simulink model "ground_test_EMF_new"  (R2024a)
settings: Solver=FixedStepAuto  StartTime=0.0  StopTime=0  FixedStep=framePeriod_s  RelTol=1e-3
undefined symbols (not defined in the file): Aircraft, aircraftIC, AircraftModel, Avphi, DiscIntNeverNeededParam, EMF, EnableFF, EnableRCHH, EnableSpeedHold, framePeriod_s, InitCond, Lv, Yv
libraries: simulink x13, simulink_extras x5
(part 2 of 3)

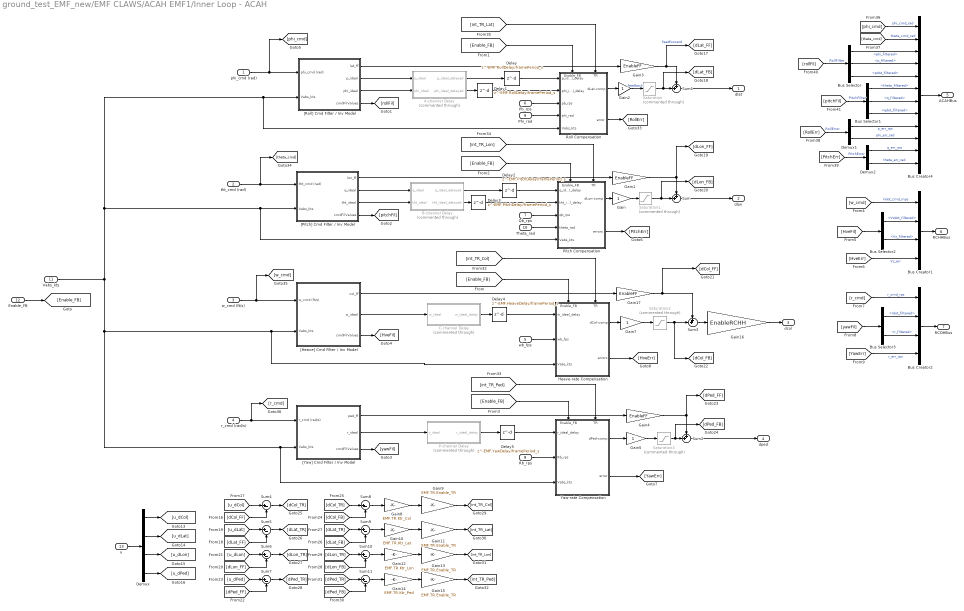
== system ground_test_EMF_new/EMF CLAWS/ACAH EMF1/Inner Loop - ACAH ==
  phi_cmd (rad) : Inport
  tht_cmd (rad) : Inport  Port=2
  w_cmd (ft/s) : Inport  Port=3
  r_cmd (rad/s) : Inport  Port=4
  wb_fps : Inport  Port=5
  Pb_rps : Inport  Port=6
  Qb_rps : Inport  Port=7
  Rb_rps : Inport  Port=8
  Phi_rad : Inport  Port=9
  Theta_rad : Inport  Port=10
  Vabs_kts : Inport  Port=11
  Enable_FB : Inport  Port=12
  u : Inport  Port=13
  A-channel Delay : Subsystem  Commented=through
  B-channel Delay : Subsystem  Commented=through
  Bus Creator1 : BusCreator  Inputs=4
  Bus Creator2 : BusCreator  Inputs=4
  Bus Creator4 : BusCreator  Inputs=12
  Bus Selector : BusSelector  OutputSignals=phi_filtered,p_filtered,pdot_filtered
  Bus Selector1 : BusSelector  OutputSignals=theta_filtered,q_filtered,qdot_filtered
  Bus Selector2 : BusSelector  OutputSignals=Vzdot_filtered,Vz_filtered
  Bus Selector3 : BusSelector  OutputSignals=rdot_filtered,r_filtered
  C-channel Delay : Subsystem  Commented=through
  Delay : Delay  DelayLength=EMF.RollDelay/framePeriod_s
  Delay1 : Delay  DelayLength=EMF.RollDelay/framePeriod_s
  Delay2 : Delay  DelayLength=EMF.PitchDelay/framePeriod_s
  Delay3 : Delay  DelayLength=EMF.PitchDelay/framePeriod_s
  Delay4 : Delay  DelayLength=EMF.HeaveDelay/framePeriod_s
  Delay5 : Delay  DelayLength=EMF.YawDelay/framePeriod_s
  Demux : Demux
  Demux1 : Demux  Outputs=2
  Demux2 : Demux  Outputs=2
  Gain{,2,5,7} (4 alike) : Gain
  Gain{1,3..4,17} (4 alike) : Gain  Gain=EnableFF
  Gain10 : Gain  Gain=EMF.TR.Ktr_Lat
  Gain{9,11,13,15} (4 alike) : Gain  Gain=EMF.TR.Enable_TR
  Gain12 : Gain  Gain=EMF.TR.Ktr_Lon
  Gain14 : Gain  Gain=EMF.TR.Ktr_Ped
  Gain16 : Gain  Gain=EnableRCHH
  Gain8 : Gain  Gain=EMF.TR.Ktr_Col
  Heave-rate Compensation : Subsystem
      settings: PortSchema="{\"entries\":[{\"content\":{\"sides\":[{\"content\":{\"connectorIds\":[\"In1\",\"In2\",\"In3\"]},\"type\":\"ConnectorPlacement.EquallySpacedRectSide\",\"uuid\":\"7252c1f8-7fe3-4075-bb5e-c3f9f1883e70\"},{\"content\":{\"connectorIds\":[\"Out1\",\"Out2\"],\"side\":\"RIGHT\"},\"type\":\"ConnectorPlacement.EquallySpacedRectSide\",\"uuid\":\"3c35276a-72f6-40d6-83e0-8018ffb9b035\"},{\"content\":{\"connectorIds\":[\"In4\",\"In5\"],\"side\":\"TOP\"},\"type\":\"ConnectorPlacement.EquallySpacedRectSide\",\"uuid\":\"6ce22a11-3d6f-44d3-856f-73f158445266\"}]},\"type\":\"ConnectorPlacement.EquallySpacedConnector\",\"uuid\":\"443ffc0d-1192-4812-a7f7-f46c9ac66e90\"}],\"packageUris\":[\"http://schema.mathworks.com/mf0/Connector/R2020b\"],\"version\":\"1.0\"}"
  P-channel Delay : Subsystem  Commented=through
  Pitch Compensation : Subsystem
      settings: PortSchema="{\"entries\":[{\"content\":{\"sides\":[{\"content\":{\"connectorIds\":[\"In1\",\"In2\",\"In3\",\"In4\",\"In5\"]},\"type\":\"ConnectorPlacement.EquallySpacedRectSide\",\"uuid\":\"45916f42-37ac-4154-8414-b45309659ed0\"},{\"content\":{\"connectorIds\":[\"Out1\",\"Out2\"],\"side\":\"RIGHT\"},\"type\":\"ConnectorPlacement.EquallySpacedRectSide\",\"uuid\":\"89f52b07-9cdc-4229-907e-581f3d5d6e1b\"},{\"content\":{\"connectorIds\":[\"In6\",\"In7\"],\"side\":\"TOP\"},\"type\":\"ConnectorPlacement.EquallySpacedRectSide\",\"uuid\":\"5e1074eb-2cc8-4130-bee4-0f8c72f9550d\"}]},\"type\":\"ConnectorPlacement.EquallySpacedConnector\",\"uuid\":\"11c4fb04-7926-4153-b42d-1368c1a6596f\"}],\"packageUris\":[\"http://schema.mathworks.com/mf0/Connector/R2020b\"],\"version\":\"1.0\"}"
  Roll Compensation : Subsystem
      settings: PortSchema="{\"entries\":[{\"content\":{\"sides\":[{\"content\":{\"connectorIds\":[\"In1\",\"In2\",\"In3\",\"In4\",\"In5\"]},\"type\":\"ConnectorPlacement.EquallySpacedRectSide\",\"uuid\":\"45916f42-37ac-4154-8414-b45309659ed0\"},{\"content\":{\"connectorIds\":[\"Out1\",\"Out2\"],\"side\":\"RIGHT\"},\"type\":\"ConnectorPlacement.EquallySpacedRectSide\",\"uuid\":\"89f52b07-9cdc-4229-907e-581f3d5d6e1b\"},{\"content\":{\"connectorIds\":[\"In6\",\"In7\"],\"side\":\"TOP\"},\"type\":\"ConnectorPlacement.EquallySpacedRectSide\",\"uuid\":\"5e1074eb-2cc8-4130-bee4-0f8c72f9550d\"}]},\"type\":\"ConnectorPlacement.EquallySpacedConnector\",\"uuid\":\"11c4fb04-7926-4153-b42d-1368c1a6596f\"}],\"packageUris\":[\"http://schema.mathworks.com/mf0/Connector/R2020b\"],\"version\":\"1.0\"}"
  Saturation : Saturate  Commented=through  UpperLimit=EMF.MaxCmd.pdot/2  LowerLimit=-EMF.MaxCmd.pdot/2
  Saturation1 : Saturate  Commented=through  UpperLimit=EMF.MaxCmd.qdot/2  LowerLimit=-EMF.MaxCmd.qdot/2
  Saturation2 : Saturate  Commented=through  UpperLimit=EMF.MaxCmd.wdot/2  LowerLimit=-EMF.MaxCmd.wdot/2
  Saturation3 : Saturate  Commented=through  UpperLimit=EMF.MaxCmd.rdot/2  LowerLimit=-EMF.MaxCmd.rdot/2
  Sum{,1..3} (4 alike) : Sum  Inputs=++|
  Sum{4..11} (8 alike) : Sum  Inputs=|+-
  Yaw-rate Compensation : Subsystem
      settings: PortSchema="{\"entries\":[{\"content\":{\"sides\":[{\"content\":{\"connectorIds\":[\"In1\",\"In2\",\"In3\"]},\"type\":\"ConnectorPlacement.EquallySpacedRectSide\",\"uuid\":\"7252c1f8-7fe3-4075-bb5e-c3f9f1883e70\"},{\"content\":{\"connectorIds\":[\"Out1\",\"Out2\"],\"side\":\"RIGHT\"},\"type\":\"ConnectorPlacement.EquallySpacedRectSide\",\"uuid\":\"3c35276a-72f6-40d6-83e0-8018ffb9b035\"},{\"content\":{\"connectorIds\":[\"In4\",\"In5\"],\"side\":\"TOP\"},\"type\":\"ConnectorPlacement.EquallySpacedRectSide\",\"uuid\":\"6ce22a11-3d6f-44d3-856f-73f158445266\"}]},\"type\":\"ConnectorPlacement.EquallySpacedConnector\",\"uuid\":\"443ffc0d-1192-4812-a7f7-f46c9ac66e90\"}],\"packageUris\":[\"http://schema.mathworks.com/mf0/Connector/R2020b\"],\"version\":\"1.0\"}"
  "[Heave] Cmd Filter / Inv Model" : Subsystem
  "[Pitch] Cmd Filter / Inv Model" : Subsystem
  "[Roll] Cmd Filter / Inv Model" : Subsystem
  "[Yaw] Cmd Filter / Inv Model" : Subsystem
  dlat : Outport
  dlon : Outport  Port=2
  dcol : Outport  Port=3
  dped : Outport  Port=4
  ACAHBus : Outport  Port=5
  RCHHBus : Outport  Port=6
  RCDHBus : Outport  Port=7
  wires:
  Gain17/1 -> [dCol_FF], Sum3/1
  Gain5/1 -> Saturation3/1
  Gain4/1 -> Sum2/1, [dPed_FF]
  Gain3/1 -> [dLat_FF], Sum1/1  "feedforward"
  Gain2/1 -> Saturation/1  "feedback"
  Gain1/1 -> [dLon_FF], Sum/1
  Gain/1 -> Saturation1/1
  wb_fps/1 -> Heave-rate Compensation/2(wb_fps)
  Rb_rps/1 -> Yaw-rate Compensation/2(Rb_rps)
  Theta_rad/1 -> Pitch Compensation/4(theta_rad)
  Qb_rps/1 -> Pitch Compensation/3(qb_rps)
  Phi_rad/1 -> Roll Compensation/4(phi_rad)
  Pb_rps/1 -> Roll Compensation/3(pb_rps)
  "[Roll] Cmd Filter / Inv Model"/1(lat_ff) -> Gain3/1
  Roll Compensation/1(dLat-comp) -> Gain2/1
  "[Pitch] Cmd Filter / Inv Model"/1(lon_ff) -> Gain1/1
  Pitch Compensation/1(dLon-comp) -> Gain/1
  w_cmd (ft/s)/1 -> [w_cmd], "[Heave] Cmd Filter / Inv Model"/1(w_cmd (ft/s))
  r_cmd (rad/s)/1 -> [r_cmd], "[Yaw] Cmd Filter / Inv Model"/1(r_cmd (rad/s))
  "[Yaw] Cmd Filter / Inv Model"/1(ped_ff) -> Gain4/1
  "[Heave] Cmd Filter / Inv Model"/1(col_ff) -> Gain17/1
  Yaw-rate Compensation/1(dPed-comp) -> Gain5/1
  Heave-rate Compensation/1(dCol-comp) -> Gain7/1
  Pitch Compensation/2(errors) -> [PitchErr]
  Yaw-rate Compensation/2(error) -> [YawErr]
  Heave-rate Compensation/2(errors) -> [HveErr]
  "[Heave] Cmd Filter / Inv Model"/3(cmdFilValues) -> [HveFil]
  "[Yaw] Cmd Filter / Inv Model"/3(cmdFilValues) -> [yawFil]
  "[Pitch] Cmd Filter / Inv Model"/4(cmdFilValues) -> [pitchFil]
  "[Roll] Cmd Filter / Inv Model"/4(cmdFilValues) -> [rollFil]
  C-channel Delay/1(w_ideal_delay) -> Delay4/1
  Sum3/1 -> Gain16/1
  "[Heave] Cmd Filter / Inv Model"/2(w_ideal) -> C-channel Delay/1(w_ideal)
  "[Yaw] Cmd Filter / Inv Model"/2(r_ideal) -> P-channel Delay/1(r_ideal)
  Sum2/1 -> dped/1
  P-channel Delay/1(r_ideal_delay) -> Delay5/1
  "[Roll] Cmd Filter / Inv Model"/3(phi_ideal) -> A-channel Delay/2(phi_ideal)
  Sum1/1 -> dlat/1
  "[Roll] Cmd Filter / Inv Model"/2(p_ideal) -> A-channel Delay/1(p_ideal)
  A-channel Delay/2(phi_ideal_delayed) -> Delay1/1
  A-channel Delay/1(p_ideal_delayed) -> Delay/1
  Sum/1 -> dlon/1
  B-channel Delay/2(tht_ideal_delayed) -> Delay3/1
  B-channel Delay/1(q_ideal_delayed) -> Delay2/1
  "[Pitch] Cmd Filter / Inv Model"/2(q_ideal) -> B-channel Delay/1(q_ideal)
  "[Pitch] Cmd Filter / Inv Model"/3(tht_ideal) -> B-channel Delay/2(tht_ideal)
  Vabs_kts/1 -> Heave-rate Compensation/3(Vabs_kts), "[Heave] Cmd Filter / Inv Model"/2(Vabs_kts), Yaw-rate Compensation/3(Vabs_kts), "[Yaw] Cmd Filter / Inv Model"/2(Vabs_kts), Pitch Compensation/5(Vabs_kts), "[Pitch] Cmd Filter / Inv Model"/2(Vabs_kts), Roll Compensation/5(Vabs_kts), "[Roll] Cmd Filter / Inv Model"/2(Vabs_kts)
  phi_cmd (rad)/1 -> [phi_cmd], "[Roll] Cmd Filter / Inv Model"/1(phi_cmd (rad))
  tht_cmd (rad)/1 -> [theta_cmd], "[Pitch] Cmd Filter / Inv Model"/1(tht_cmd (rad))
  Delay1/1 -> Roll Compensation/2(phi_ideal_delay)
  Delay/1 -> Roll Compensation/1(p_ideal_delay)
  Delay3/1 -> Pitch Compensation/2(tht_ideal_delay)
  Delay2/1 -> Pitch Compensation/1(q_ideal_delay)
  Delay4/1 -> Heave-rate Compensation/1(w_ideal_delay)
  Delay5/1 -> Yaw-rate Compensation/1(r_ideal_delay)
  Enable_FB/1 -> [Enable_FB]
  [Enable_FB] -> Heave-rate Compensation/4(Enable_FB)
  [Enable_FB] -> Roll Compensation/6(Enable_FB)
  [Enable_FB] -> Pitch Compensation/6(Enable_FB)
  [Enable_FB] -> Yaw-rate Compensation/4(Enable_FB)
  Gain7/1 -> Saturation2/1
  Saturation/1 -> [dLat_FB], Sum1/2
  Saturation1/1 -> [dLon_FB], Sum/2
  Saturation3/1 -> [dPed_FB], Sum2/2
  u/1 -> Demux/1
  Demux/1 -> [u_dCol]
  Demux/4 -> [u_dPed]
  Demux/3 -> [u_dLon]
  Demux/2 -> [u_dLat]
  [u_dCol] -> Sum4/1
  [dCol_FF] -> Sum4/2
  Sum4/1 -> [dCol_TR]
  Sum5/1 -> [dLat_TR]
  [dLat_FF] -> Sum5/2
  [u_dLat] -> Sum5/1
  [u_dLon] -> Sum6/1
  [dLon_FF] -> Sum6/2
  Sum6/1 -> [dLon_TR]
  Sum7/1 -> [dPed_TR]
  [dPed_FF] -> Sum7/2
  [u_dPed] -> Sum7/1
  Sum8/1 -> Gain8/1
  [dCol_FB] -> Sum8/2
  [dCol_TR] -> Sum8/1
  Gain8/1 -> Gain9/1
  Gain9/1 -> [int_TR_Col]
  Gain11/1 -> [int_TR_Lat]
  Gain10/1 -> Gain11/1
  [dLat_TR] -> Sum9/1
  [dLat_FB] -> Sum9/2
  Sum9/1 -> Gain10/1
  Sum10/1 -> Gain12/1
  [dLon_FB] -> Sum10/2
  [dLon_TR] -> Sum10/1
  Gain12/1 -> Gain13/1
  Gain13/1 -> [int_TR_Lon]
  Gain15/1 -> [int_TR_Ped]
  Gain14/1 -> Gain15/1
  [dPed_TR] -> Sum11/1
  [dPed_FB] -> Sum11/2
  Sum11/1 -> Gain14/1
  [int_TR_Col] -> Heave-rate Compensation/5(TR)
  [int_TR_Ped] -> Yaw-rate Compensation/5(TR)
  [int_TR_Lon] -> Pitch Compensation/7(TR)
  [int_TR_Lat] -> Roll Compensation/7(TR)
  Saturation2/1 -> [dCol_FB], Sum3/2
  Gain16/1 -> dcol/1
  Roll Compensation/2(error) -> [RollErr]
  Bus Creator4/1 -> ACAHBus/1
  [phi_cmd] -> Bus Creator4/1  "phi_cmd_rad"
  [theta_cmd] -> Bus Creator4/2  "theta_cmd_rad"
  [rollFil] -> Bus Selector/1  "RollFilter"
  [pitchFil] -> Bus Selector1/1  "PitchFilter"
  Bus Selector/2 -> Bus Creator4/4  "<p_filtered>"
  Bus Selector/1 -> Bus Creator4/3  "<phi_filtered>"
  Bus Selector/3 -> Bus Creator4/5  "<pdot_filtered>"
  Bus Selector1/1 -> Bus Creator4/6  "<theta_filtered>"
  Bus Selector1/2 -> Bus Creator4/7  "<q_filtered>"
  Bus Selector1/3 -> Bus Creator4/8  "<qdot_filtered>"
  [RollErr] -> Demux1/1  "RollError"
  [PitchErr] -> Demux2/1  "PitchError"
  Demux2/2 -> Bus Creator4/12  "theta_err_rad"
  Demux2/1 -> Bus Creator4/11  "q_err_rps"
  Demux1/1 -> Bus Creator4/9  "p_err_rps"
  Demux1/2 -> Bus Creator4/10  "phi_err_rad"
  Bus Creator1/1 -> RCHHBus/1
  [w_cmd] -> Bus Creator1/1  "hdot_cmd_mps"
  [HveFil] -> Bus Selector2/1
  Bus Selector2/2 -> Bus Creator1/3  "<Vz_filtered>"
  Bus Selector2/1 -> Bus Creator1/2  "<Vzdot_filtered>"
  [HveErr] -> Bus Creator1/4  "Vz_err"
  [YawErr] -> Bus Creator2/4  "r_err_rps"
  Bus Selector3/1 -> Bus Creator2/2  "<rdot_filtered>"
  Bus Selector3/2 -> Bus Creator2/3  "<r_filtered>"
  [yawFil] -> Bus Selector3/1
  [r_cmd] -> Bus Creator2/1  "r_cmd_rps"
  Bus Creator2/1 -> RCDHBus/1

== system ground_test_EMF_new/EMF CLAWS/ACAH EMF1/Mixer ==
  ControlMoments : Inport
  Constant : Constant  Value=EMF.Mixer(:,:,1)
  Matrix Multiply : Product  Multiplication=Matrix(*)
  Rotor Speeds : Outport
  wires:
  Constant/1 -> Matrix Multiply/1
  ControlMoments/1 -> Matrix Multiply/2
  Matrix Multiply/1 -> Rotor Speeds/1  "Rotor Speeds"

== system ground_test_EMF_new/EMF CLAWS/ACAH EMF1/OnGroundController ==
  cmdsACT : Inport
  Get ACAH Commands1 : Subsystem
      settings: PortSchema="{\"entries\":[{\"content\":{\"sides\":[{\"content\":{\"connectorIds\":[\"In1\"]},\"type\":\"ConnectorPlacement.EquallySpacedRectSide\",\"uuid\":\"7c65b894-e97e-426b-b3a6-5e2b2b7aa780\"},{\"content\":{\"connectorIds\":[\"Out1\"],\"side\":\"RIGHT\"},\"type\":\"ConnectorPlacement.EquallySpacedRectSide\",\"uuid\":\"da5e6856-a2cd-4302-9f49-e9c1cc422564\"},{\"content\":{\"connectorIds\":[\"Out2\"],\"side\":\"TOP\"},\"type\":\"ConnectorPlacement.EquallySpacedRectSide\",\"uuid\":\"a744aea1-4523-47bd-90bf-604bddb972da\"}]},\"type\":\"ConnectorPlacement.EquallySpacedConnector\",\"uuid\":\"254b2f3c-23c2-4cd5-a42e-cd931c0875f5\"}],\"packageUris\":[\"http://schema.mathworks.com/mf0/Connector/R2020b\"],\"version\":\"1.0\"}"
  OL rotor speeds from throttle : Subsystem  Commented=through
  TrimOmegas_OL : Outport
  CmdMoments_Ground : Outport  Port=2
  wires:
  cmdsACT/1 -> Get ACAH Commands1/1(StickInputs)
  Get ACAH Commands1/1(cmdsACAH) -> CmdMoments_Ground/1
  Get ACAH Commands1/2(throttleOmega) -> OL rotor speeds from throttle/1(throttleOmega)
  OL rotor speeds from throttle/1(Omegas_rps) -> TrimOmegas_OL/1

== system ground_test_EMF_new/EMF CLAWS/ACAH EMF1/Rate Saturation ==
  dlat : Inport
  dlon : Inport  Port=2
  dcol : Inport  Port=3
  dped : Inport  Port=4
  Compare To Constant1 : simulink/Logic and Bit Operations/Compare To Constant  relop=<  const=-EMF.MaxCmd.qdot  OutDataTypeStr=boolean
  Compare To Constant2 : simulink/Logic and Bit Operations/Compare To Constant  relop=>  const=EMF.MaxCmd.qdot  OutDataTypeStr=boolean
  Compare To Constant3 : simulink/Logic and Bit Operations/Compare To Constant  relop=<  const=-EMF.MaxCmd.wdot  OutDataTypeStr=boolean
  Compare To Constant4 : simulink/Logic and Bit Operations/Compare To Constant  relop=>  const=EMF.MaxCmd.wdot  OutDataTypeStr=boolean
  Compare To Constant5 : simulink/Logic and Bit Operations/Compare To Constant  relop=<  const=-EMF.MaxCmd.rdot  OutDataTypeStr=boolean
  Compare To Constant6 : simulink/Logic and Bit Operations/Compare To Constant  relop=>  const=EMF.MaxCmd.rdot  OutDataTypeStr=boolean
  Compare To Constant7 : simulink/Logic and Bit Operations/Compare To Constant  relop=<  const=-EMF.MaxCmd.pdot  OutDataTypeStr=boolean
  Compare To Constant8 : simulink/Logic and Bit Operations/Compare To Constant  relop=>  const=EMF.MaxCmd.pdot  OutDataTypeStr=boolean
  Logical Operator{1..4} (4 alike) : Logic  Operator=OR  AllPortsSameDT=off  OutDataTypeStr=boolean
  Mux : Mux
  Saturation : Saturate  UpperLimit=EMF.MaxCmd.pdot  LowerLimit=-EMF.MaxCmd.pdot
  Saturation1 : Saturate  UpperLimit=EMF.MaxCmd.qdot  LowerLimit=-EMF.MaxCmd.qdot
  Saturation2 : Saturate  UpperLimit=EMF.MaxCmd.wdot  LowerLimit=-EMF.MaxCmd.wdot
  Saturation3 : Saturate  UpperLimit=EMF.MaxCmd.rdot  LowerLimit=-EMF.MaxCmd.rdot
  dcol sat : Outport
  dlat sat : Outport  Port=2
  dlon sat : Outport  Port=3
  dped sat : Outport  Port=4
  Flag : Outport  Port=5
  wires:
  Saturation3/1 -> dped sat/1
  Saturation1/1 -> dlon sat/1
  Saturation/1 -> dlat sat/1
  dlat/1 -> Compare To Constant8/1, Compare To Constant7/1, Saturation/1
  Saturation2/1 -> dcol sat/1
  Compare To Constant7/1 -> Logical Operator4/2
  Compare To Constant8/1 -> Logical Operator4/1
  Logical Operator4/1 -> Mux/1
  Logical Operator1/1 -> Mux/2
  Compare To Constant2/1 -> Logical Operator1/1
  Compare To Constant1/1 -> Logical Operator1/2
  dlon/1 -> Compare To Constant2/1, Compare To Constant1/1, Saturation1/1
  dcol/1 -> Compare To Constant3/1, Compare To Constant4/1, Saturation2/1
  Compare To Constant3/1 -> Logical Operator2/2
  Compare To Constant4/1 -> Logical Operator2/1
  Logical Operator2/1 -> Mux/3
  Logical Operator3/1 -> Mux/4
  Compare To Constant6/1 -> Logical Operator3/1
  Compare To Constant5/1 -> Logical Operator3/2
  dped/1 -> Saturation3/1, Compare To Constant6/1, Compare To Constant5/1
  Mux/1 -> Flag/1

== system ground_test_EMF_new/EMF CLAWS/ACAH EMF1/Remap Rotor Speeds to PWM ==
  Rotor Speeds : Inport
  Constant1 : Constant  Value=AircraftModel.MinOmegaLimit
  Constant2 : Constant  Value=AircraftModel.MaxOmegaLimit
  Constant3 : Constant  Value=AircraftModel.MinPWMLimit*ones(1,4)
  Constant4 : Constant  Value=AircraftModel.MaxPWMLimit*ones(4,1)
  Rotor Speed Saturation : Subsystem
  remap : MATLAB Function  TreatAsAtomicUnit=on
  PWM_int16 : Outport
  tag scope: OmSatFlag=global
  wires:
  Rotor Speed Saturation/2(Saturated Rotor Speeds) -> remap/1(norm_in)
  Rotor Speed Saturation/1(OmegaSaturationFlags) -> [OmSatFlag]
  Constant2/1 -> remap/3(in_max)
  remap/1(raw_out) -> PWM_int16/1  "PWM_cont"
  Constant4/1 -> remap/5(out_max)
  Constant1/1 -> remap/2(in_min)
  Constant3/1 -> remap/4(out_min)
  Rotor Speeds/1 -> Rotor Speed Saturation/1(Rotor Speeds)

== system ground_test_EMF_new/EMF CLAWS/ACAH EMF1/Subsystem ==
  StateBus : Inport
  Add : Sum  Inputs=+++
  Bus Selector1 : BusSelector  OutputSignals=u_fdbk_mps,v_fdbk_mps,w_fdbk_mps
  Gain : Gain  Gain=0
  Sqrt : Sqrt
  Square : Math  Operator=square
  Square1 : Math  Operator=square
  Square2 : Math  Operator=square
  fps_to_kts : Gain  Gain=0.592484
  Vabs_kts : Outport
  wires:
  Square1/1 -> Add/2
  Bus Selector1/3 -> Square2/1  "<w_fdbk_mps>"
  StateBus/1 -> Bus Selector1/1
  Add/1 -> Sqrt/1
  Square/1 -> Add/1
  Bus Selector1/1 -> Square/1  "<u_fdbk_mps>"
  Bus Selector1/2 -> Gain/1  "<v_fdbk_mps>"
  Sqrt/1 -> fps_to_kts/1
  Square2/1 -> Add/3
  Gain/1 -> Square1/1
  fps_to_kts/1 -> Vabs_kts/1

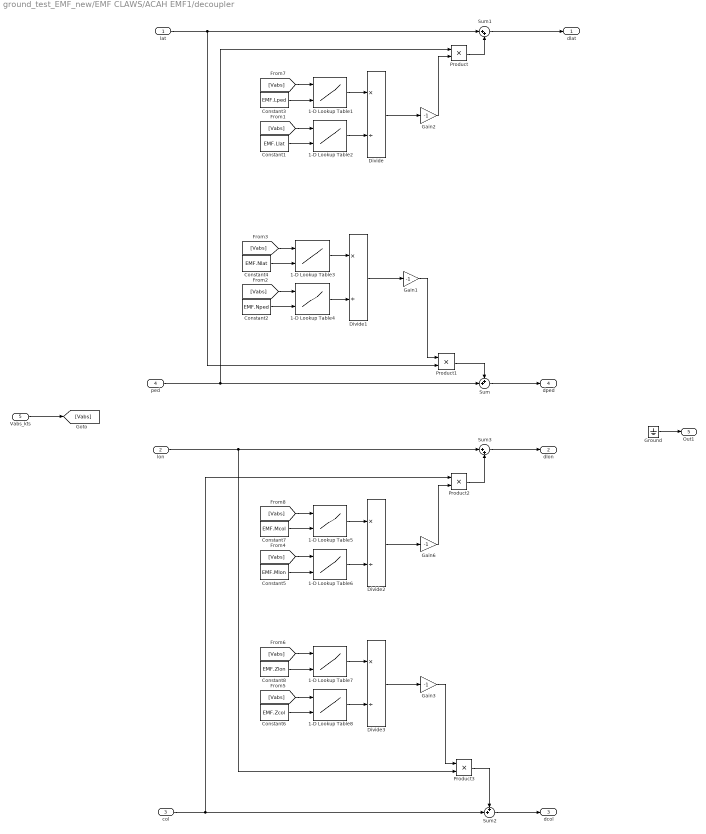
== system ground_test_EMF_new/EMF CLAWS/ACAH EMF1/decoupler ==
  lat : Inport
  lon : Inport  Port=2
  col : Inport  Port=3
  ped : Inport  Port=4
  Vabs_kts : Inport  Port=5
  1-D Lookup Table{1..8} (8 alike) : Lookup_n-D  NumberOfTableDimensions=1  BreakpointsForDimension1=EMF.VTAB  BeginIndexSearchUsingPreviousIndexResult=on  TableSource=Input port  Table=tanh([-5:5])  ExtrapMethod=Clip  InternalRulePriority=Speed  RndMeth=Simplest
      settings: InputPortMap=u0,p221
  Constant1 : Constant  Value=EMF.Llat
  Constant2 : Constant  Value=EMF.Nped
  Constant3 : Constant  Value=EMF.Lped
  Constant4 : Constant  Value=EMF.Nlat
  Constant5 : Constant  Value=EMF.Mlon
  Constant6 : Constant  Value=EMF.Zcol
  Constant7 : Constant  Value=EMF.Mcol
  Constant8 : Constant  Value=EMF.Zlon
  Divide{,1..3} (4 alike) : Product  Inputs=*/
  Gain{1..3,6} (4 alike) : Gain  Gain=-1
  Ground : Ground
  Product{,1..3} (4 alike) : Product
  Sum : Sum  Inputs=++|
  Sum1 : Sum  Inputs=|++
  Sum2 : Sum  Inputs=++|
  Sum3 : Sum  Inputs=|++
  dlat : Outport
  dlon : Outport  Port=2
  dcol : Outport  Port=3
  dped : Outport  Port=4
  Out1 : Outport  Port=5
  wires:
  Vabs_kts/1 -> [Vabs]
  Product3/1 -> Sum2/1
  Product2/1 -> Sum3/2
  Constant7/1 -> 1-D Lookup Table5/2
  [Vabs] -> 1-D Lookup Table5/1
  [Vabs] -> 1-D Lookup Table6/1
  Constant5/1 -> 1-D Lookup Table6/2
  1-D Lookup Table6/1 -> Divide2/2
  1-D Lookup Table5/1 -> Divide2/1
  Divide2/1 -> Gain6/1
  Gain6/1 -> Product2/2
  Gain3/1 -> Product3/1
  Divide3/1 -> Gain3/1
  1-D Lookup Table7/1 -> Divide3/1
  1-D Lookup Table8/1 -> Divide3/2
  Constant6/1 -> 1-D Lookup Table8/2
  [Vabs] -> 1-D Lookup Table8/1
  [Vabs] -> 1-D Lookup Table7/1
  Constant8/1 -> 1-D Lookup Table7/2
  Product1/1 -> Sum/1
  Constant4/1 -> 1-D Lookup Table3/2
  [Vabs] -> 1-D Lookup Table3/1
  [Vabs] -> 1-D Lookup Table4/1
  Constant2/1 -> 1-D Lookup Table4/2
  1-D Lookup Table4/1 -> Divide1/2
  1-D Lookup Table3/1 -> Divide1/1
  Divide1/1 -> Gain1/1
  Gain1/1 -> Product1/1
  Gain2/1 -> Product/2
  Product/1 -> Sum1/2
  Divide/1 -> Gain2/1
  1-D Lookup Table1/1 -> Divide/1
  1-D Lookup Table2/1 -> Divide/2
  Constant1/1 -> 1-D Lookup Table2/2
  [Vabs] -> 1-D Lookup Table2/1
  [Vabs] -> 1-D Lookup Table1/1
  Constant3/1 -> 1-D Lookup Table1/2
  Sum3/1 -> dlon/1
  Sum2/1 -> dcol/1
  Sum1/1 -> dlat/1
  ped/1 -> Sum/2, Product/1
  lat/1 -> Sum1/1, Product1/2
  Sum/1 -> dped/1
  col/1 -> Product2/1, Sum2/2
  lon/1 -> Product3/2, Sum3/1
  Ground/1 -> Out1/1

== system ground_test_EMF_new/EMF CLAWS/ACAH EMF1/Inner Loop - ACAH/A-channel Delay ==
  p_ideal : Inport
  phi_ideal : Inport  Port=2
  Constant : Constant  Value=EMF.tauf
  Demux : Demux  Outputs=2
  Divide : Product  Inputs=*/
  Integrator : Integrator
  Mux : Mux  Inputs=2
  Sum : Sum  Inputs=|+-
  p_ideal_delayed : Outport
  phi_ideal_delayed : Outport  Port=2
  wires:
  Demux/2 -> phi_ideal_delayed/1
  Demux/1 -> p_ideal_delayed/1
  phi_ideal/1 -> Mux/2
  p_ideal/1 -> Mux/1
  Mux/1 -> Sum/1
  Constant/1 -> Divide/2
  Divide/1 -> Integrator/1
  Sum/1 -> Divide/1
  Integrator/1 -> Demux/1, Sum/2

== system ground_test_EMF_new/EMF CLAWS/ACAH EMF1/Inner Loop - ACAH/B-channel Delay ==
  q_ideal : Inport
  tht_ideal : Inport  Port=2
  Constant : Constant  Value=EMF.tauf
  Demux : Demux  Outputs=2
  Divide : Product  Inputs=*/
  Integrator : Integrator
  Mux : Mux  Inputs=2
  Sum : Sum  Inputs=|+-
  q_ideal_delayed : Outport
  tht_ideal_delayed : Outport  Port=2
  wires:
  Demux/2 -> tht_ideal_delayed/1
  Demux/1 -> q_ideal_delayed/1
  tht_ideal/1 -> Mux/2
  q_ideal/1 -> Mux/1
  Mux/1 -> Sum/1
  Constant/1 -> Divide/2
  Divide/1 -> Integrator/1
  Sum/1 -> Divide/1
  Integrator/1 -> Demux/1, Sum/2

== system ground_test_EMF_new/EMF CLAWS/ACAH EMF1/Inner Loop - ACAH/C-channel Delay ==
  w_ideal : Inport
  Constant : Constant  Value=EMF.tauf
  Divide : Product  Inputs=*/
  Integrator : Integrator
  Sum : Sum  Inputs=|+-
  w_ideal_delay : Outport
  wires:
  w_ideal/1 -> Sum/1
  Constant/1 -> Divide/2
  Divide/1 -> Integrator/1
  Sum/1 -> Divide/1
  Integrator/1 -> w_ideal_delay/1, Sum/2

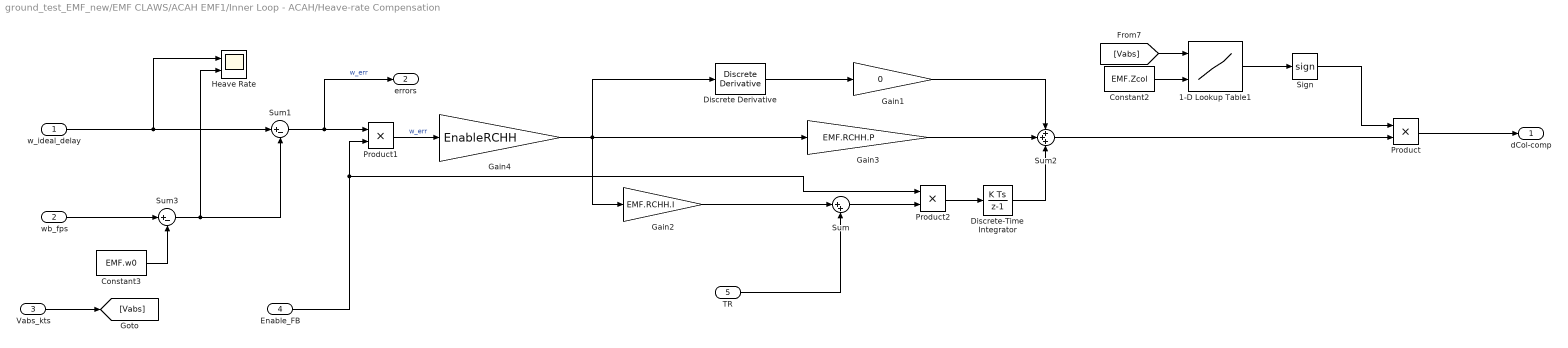
== system ground_test_EMF_new/EMF CLAWS/ACAH EMF1/Inner Loop - ACAH/Heave-rate Compensation ==
  w_ideal_delay : Inport
  wb_fps : Inport  Port=2
  Vabs_kts : Inport  Port=3
  Enable_FB : Inport  Port=4
  TR : Inport  Port=5
  1-D Lookup Table1 : Lookup_n-D  NumberOfTableDimensions=1  BreakpointsForDimension1=EMF.VTAB  BeginIndexSearchUsingPreviousIndexResult=on  TableSource=Input port  Table=tanh([-5:5])  ExtrapMethod=Clip  InternalRulePriority=Speed  RndMeth=Simplest
      settings: InputPortMap=u0,p221
  Constant2 : Constant  Value=EMF.Zcol
  Constant3 : Constant  Value=EMF.w0
  Discrete Derivative : simulink/Discrete/Discrete Derivative  gainval=1.0  ICPrevScaledInput=0.0  OutMin=[]  OutMax=[]  OutDataType=fixdt(1, 16)  OutScaling=2^-10  DoSatur=off
  Discrete-Time Integrator : DiscreteIntegrator  SampleTime=-1  ICPrevOutput=DiscIntNeverNeededParam  ICPrevScaledInput=DiscIntNeverNeededParam
  Gain1 : Gain  Gain=0
  Gain2 : Gain  Gain=EMF.RCHH.I
  Gain3 : Gain  Gain=EMF.RCHH.P
  Gain4 : Gain  Gain=EnableRCHH
  Heave Rate : Scope  NumInputPorts=2
  Product : Product
  Product1 : Product
  Product2 : Product
  Sign : Signum
  Sum : Sum  Inputs=|++
  Sum1 : Sum  Inputs=|+-
  Sum2 : Sum  Inputs=+++
  Sum3 : Sum  Inputs=|+-
  dCol-comp : Outport
  errors : Outport  Port=2
  wires:
  Gain3/1 -> Sum2/2
  Sum/1 -> Product2/2
  wb_fps/1 -> Sum3/1
  Sign/1 -> Product/1
  1-D Lookup Table1/1 -> Sign/1
  Product/1 -> dCol-comp/1
  Discrete Derivative/1 -> Gain1/1
  Product1/1 -> Gain4/1  "w_err"
  Sum2/1 -> Product/2
  Gain1/1 -> Sum2/1
  w_ideal_delay/1 -> Heave Rate/1, Sum1/1
  [Vabs] -> 1-D Lookup Table1/1
  Constant2/1 -> 1-D Lookup Table1/2
  Vabs_kts/1 -> [Vabs]
  Sum3/1 -> Heave Rate/2, Sum1/2
  Constant3/1 -> Sum3/2
  Sum1/1 -> errors/1, Product1/1  "w_err"
  Enable_FB/1 -> Product2/1, Product1/2
  Discrete-Time Integrator/1 -> Sum2/3
  Product2/1 -> Discrete-Time Integrator/1
  Gain2/1 -> Sum/1
  TR/1 -> Sum/2
  Gain4/1 -> Discrete Derivative/1, Gain3/1, Gain2/1

== system ground_test_EMF_new/EMF CLAWS/ACAH EMF1/Inner Loop - ACAH/P-channel Delay ==
  r_ideal : Inport
  Constant : Constant  Value=EMF.tauf
  Divide : Product  Inputs=*/
  Integrator : Integrator
  Sum : Sum  Inputs=|+-
  r_ideal_delay : Outport
  wires:
  Divide/1 -> Integrator/1
  r_ideal/1 -> Sum/1
  Integrator/1 -> Sum/2, r_ideal_delay/1
  Constant/1 -> Divide/2
  Sum/1 -> Divide/1

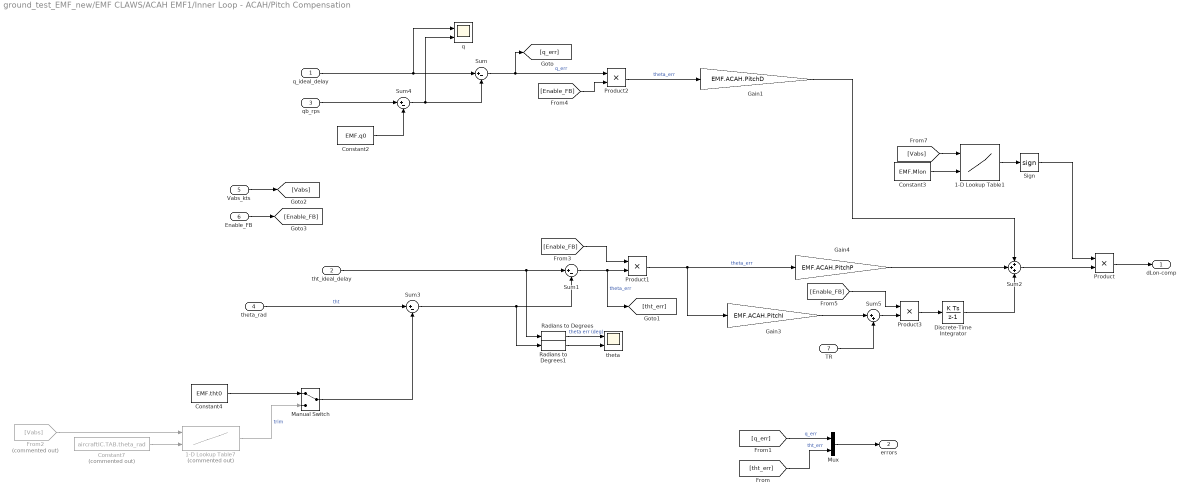
== system ground_test_EMF_new/EMF CLAWS/ACAH EMF1/Inner Loop - ACAH/Pitch Compensation ==
  q_ideal_delay : Inport
  tht_ideal_delay : Inport  Port=2
  qb_rps : Inport  Port=3
  theta_rad : Inport  Port=4
  Vabs_kts : Inport  Port=5
  Enable_FB : Inport  Port=6
  TR : Inport  Port=7
  1-D Lookup Table1 : Lookup_n-D  NumberOfTableDimensions=1  BreakpointsForDimension1=EMF.VTAB  BeginIndexSearchUsingPreviousIndexResult=on  TableSource=Input port  Table=tanh([-5:5])  ExtrapMethod=Clip  InternalRulePriority=Speed  RndMeth=Simplest
      settings: InputPortMap=u0,p221
  1-D Lookup Table7 : Lookup_n-D  Commented=on  NumberOfTableDimensions=1  BreakpointsForDimension1=EMF.VTAB  BeginIndexSearchUsingPreviousIndexResult=on  TableSource=Input port  Table=tanh([-5:5])  ExtrapMethod=Clip  InternalRulePriority=Speed  RndMeth=Simplest
      settings: InputPortMap=u0,p221
  Constant2 : Constant  Value=EMF.q0
  Constant3 : Constant  Value=EMF.Mlon
  Constant4 : Constant  Value=EMF.tht0
  Constant7 : Constant  Commented=on  Value=aircraftIC.TAB.theta_rad
  Discrete-Time Integrator : DiscreteIntegrator  SampleTime=-1  ICPrevOutput=DiscIntNeverNeededParam  ICPrevScaledInput=DiscIntNeverNeededParam
  From2 : From  Commented=on  GotoTag=Vabs
  Gain1 : Gain  Gain=EMF.ACAH.PitchD
  Gain3 : Gain  Gain=EMF.ACAH.PitchI
  Gain4 : Gain  Gain=EMF.ACAH.PitchP
  Manual Switch : ManualSwitch
  Mux : Mux  Inputs=2
  Product{,1..3} (4 alike) : Product
  Radians to Degrees : simulink_extras/Transformations/Radians to Degrees
  Radians to Degrees1 : simulink_extras/Transformations/Radians to Degrees
  Sign : Signum
  Sum{,1,3..4} (4 alike) : Sum  Inputs=|+-
  Sum2 : Sum  Inputs=+++
  Sum5 : Sum  Inputs=|++
  q : Scope  NumInputPorts=2
  theta : Scope  NumInputPorts=2
  dLon-comp : Outport
  errors : Outport  Port=2
  wires:
  Gain4/1 -> Sum2/2
  Sign/1 -> Product/1
  Product/1 -> dLon-comp/1
  Gain1/1 -> Sum2/1
  [q_err] -> Mux/1  "q_err"
  Mux/1 -> errors/1
  [tht_err] -> Mux/2  "tht_err"
  Sum/1 -> Product2/1, [q_err]  "q_err"
  Product1/1 -> Gain3/1, Gain4/1  "theta_err"
  q_ideal_delay/1 -> Sum/1, q/1
  qb_rps/1 -> Sum4/1
  Sum4/1 -> Sum/2, q/2
  Constant2/1 -> Sum4/2
  [Vabs] -> 1-D Lookup Table1/1
  Constant3/1 -> 1-D Lookup Table1/2
  1-D Lookup Table1/1 -> Sign/1
  Vabs_kts/1 -> [Vabs]
  Radians to Degrees/1 -> theta/1  "theta err (deg)"
  Radians to Degrees1/1 -> theta/2
  Constant7/1 -> 1-D Lookup Table7/2
  Constant4/1 -> Manual Switch/1
  Sum3/1 -> Sum1/2, Radians to Degrees1/1
  From2/1 -> 1-D Lookup Table7/1
  theta_rad/1 -> Sum3/1  "tht"
  1-D Lookup Table7/1 -> Manual Switch/2  "trim"
  Sum5/1 -> Product3/2
  tht_ideal_delay/1 -> Sum1/1, Radians to Degrees/1
  Sum2/1 -> Product/2
  Manual Switch/1 -> Sum3/2
  Sum1/1 -> [tht_err], Product1/2  "theta_err"
  Enable_FB/1 -> [Enable_FB]
  [Enable_FB] -> Product1/1
  Product2/1 -> Gain1/1  "theta_err"
  [Enable_FB] -> Product2/2
  Discrete-Time Integrator/1 -> Sum2/3
  Product3/1 -> Discrete-Time Integrator/1
  [Enable_FB] -> Product3/1
  Gain3/1 -> Sum5/1
  TR/1 -> Sum5/2

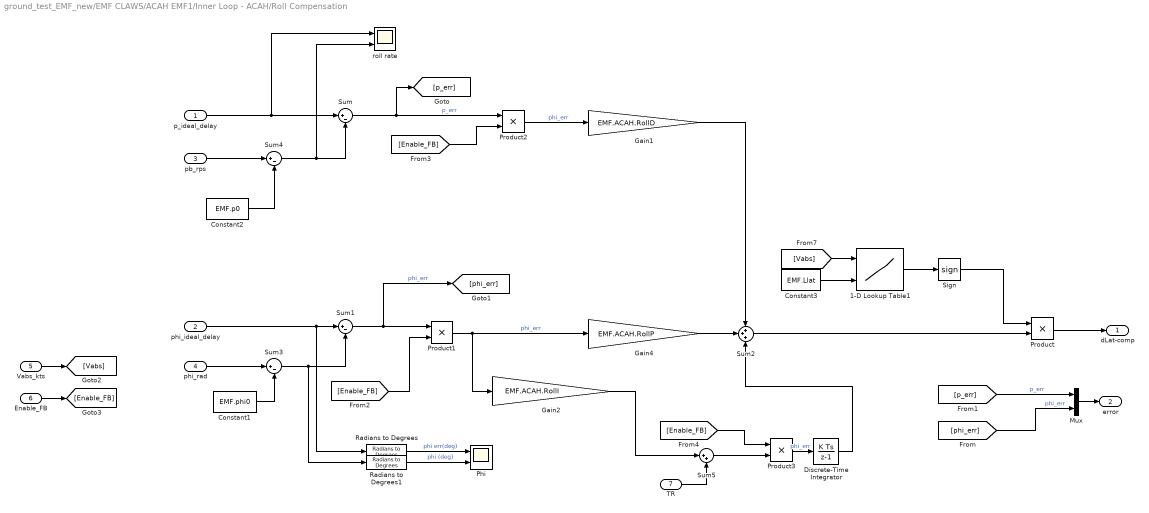
== system ground_test_EMF_new/EMF CLAWS/ACAH EMF1/Inner Loop - ACAH/Roll Compensation ==
  p_ideal_delay : Inport
  phi_ideal_delay : Inport  Port=2
  pb_rps : Inport  Port=3
  phi_rad : Inport  Port=4
  Vabs_kts : Inport  Port=5
  Enable_FB : Inport  Port=6
  TR : Inport  Port=7
  1-D Lookup Table1 : Lookup_n-D  NumberOfTableDimensions=1  BreakpointsForDimension1=EMF.VTAB  BeginIndexSearchUsingPreviousIndexResult=on  TableSource=Input port  Table=tanh([-5:5])  ExtrapMethod=Clip  InternalRulePriority=Speed  RndMeth=Simplest
      settings: InputPortMap=u0,p221
  Constant1 : Constant  Value=EMF.phi0
  Constant2 : Constant  Value=EMF.p0
  Constant3 : Constant  Value=EMF.Llat
  Discrete-Time Integrator : DiscreteIntegrator  SampleTime=-1  ICPrevOutput=DiscIntNeverNeededParam  ICPrevScaledInput=DiscIntNeverNeededParam
  Gain1 : Gain  Gain=EMF.ACAH.RollD
  Gain2 : Gain  Gain=EMF.ACAH.RollI
  Gain4 : Gain  Gain=EMF.ACAH.RollP
  Mux : Mux  Inputs=2
  Phi : Scope  NumInputPorts=2
  Product{,1..3} (4 alike) : Product
  Radians to Degrees : simulink_extras/Transformations/Radians to Degrees
  Radians to Degrees1 : simulink_extras/Transformations/Radians to Degrees
  Sign : Signum
  Sum{,1,3..4} (4 alike) : Sum  Inputs=|+-
  Sum2 : Sum  Inputs=+++
  Sum5 : Sum  Inputs=|++
  roll rate : Scope  NumInputPorts=2
  dLat-comp : Outport
  error : Outport  Port=2
  wires:
  Gain4/1 -> Sum2/2
  Sum2/1 -> Product/2
  Sign/1 -> Product/1
  Product/1 -> dLat-comp/1
  [phi_err] -> Mux/2  "phi_err"
  phi_ideal_delay/1 -> Sum1/1, Radians to Degrees/1
  phi_rad/1 -> Sum3/1
  Sum/1 -> [p_err], Product2/1  "p_err"
  Gain1/1 -> Sum2/1
  Product1/1 -> Gain2/1, Gain4/1  "phi_err"
  p_ideal_delay/1 -> Sum/1, roll rate/1
  Sum3/1 -> Radians to Degrees1/1, Sum1/2
  Constant1/1 -> Sum3/2
  Sum4/1 -> Sum/2, roll rate/2
  Constant2/1 -> Sum4/2
  pb_rps/1 -> Sum4/1
  [Vabs] -> 1-D Lookup Table1/1
  Constant3/1 -> 1-D Lookup Table1/2
  Vabs_kts/1 -> [Vabs]
  1-D Lookup Table1/1 -> Sign/1
  Sum5/1 -> Product3/2
  Radians to Degrees/1 -> Phi/1  "phi err(deg)"
  Radians to Degrees1/1 -> Phi/2  "phi (deg)"
  Enable_FB/1 -> [Enable_FB]
  Sum1/1 -> [phi_err], Product1/1  "phi_err"
  [Enable_FB] -> Product1/2
  Product2/1 -> Gain1/1  "phi_err"
  [Enable_FB] -> Product2/2
  Discrete-Time Integrator/1 -> Sum2/3
  Product3/1 -> Discrete-Time Integrator/1  "phi_err"
  [Enable_FB] -> Product3/1
  Gain2/1 -> Sum5/1
  TR/1 -> Sum5/2
  Mux/1 -> error/1
  [p_err] -> Mux/1  "p_err"

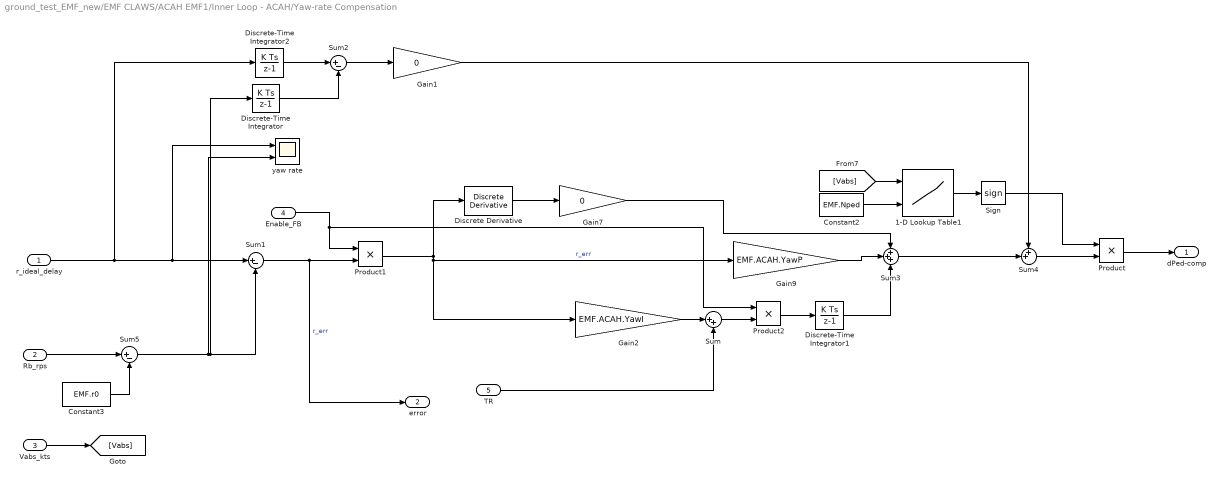
== system ground_test_EMF_new/EMF CLAWS/ACAH EMF1/Inner Loop - ACAH/Yaw-rate Compensation ==
  r_ideal_delay : Inport
  Rb_rps : Inport  Port=2
  Vabs_kts : Inport  Port=3
  Enable_FB : Inport  Port=4
  TR : Inport  Port=5
  1-D Lookup Table1 : Lookup_n-D  NumberOfTableDimensions=1  BreakpointsForDimension1=EMF.VTAB  BeginIndexSearchUsingPreviousIndexResult=on  TableSource=Input port  Table=tanh([-5:5])  ExtrapMethod=Clip  InternalRulePriority=Speed  RndMeth=Simplest
      settings: InputPortMap=u0,p221
  Constant2 : Constant  Value=EMF.Nped
  Constant3 : Constant  Value=EMF.r0
  Discrete Derivative : simulink/Discrete/Discrete Derivative  gainval=1.0  ICPrevScaledInput=0.0  OutMin=[]  OutMax=[]  OutDataType=fixdt(1, 16)  OutScaling=2^-10  DoSatur=off
  Discrete-Time Integrator : DiscreteIntegrator  SampleTime=-1  ICPrevOutput=DiscIntNeverNeededParam  ICPrevScaledInput=DiscIntNeverNeededParam
  Discrete-Time Integrator1 : DiscreteIntegrator  SampleTime=-1  ICPrevOutput=DiscIntNeverNeededParam  ICPrevScaledInput=DiscIntNeverNeededParam
  Discrete-Time Integrator2 : DiscreteIntegrator  SampleTime=-1  ICPrevOutput=DiscIntNeverNeededParam  ICPrevScaledInput=DiscIntNeverNeededParam
  Gain1 : Gain  Gain=0
  Gain2 : Gain  Gain=EMF.ACAH.YawI
  Gain7 : Gain  Gain=0
  Gain9 : Gain  Gain=EMF.ACAH.YawP
  Product : Product
  Product1 : Product
  Product2 : Product
  Sign : Signum
  Sum : Sum  Inputs=|++
  Sum1 : Sum  Inputs=|+-
  Sum2 : Sum  Inputs=|+-
  Sum3 : Sum  Inputs=+++
  Sum4 : Sum  Inputs=++|
  Sum5 : Sum  Inputs=|+-
  yaw rate : Scope  NumInputPorts=2
  dPed-comp : Outport
  error : Outport  Port=2
  wires:
  Product1/1 -> Discrete Derivative/1, Gain2/1, Gain9/1  "r_err"
  Discrete Derivative/1 -> Gain7/1
  Gain7/1 -> Sum3/1
  Gain9/1 -> Sum3/2
  Sum/1 -> Product2/2
  Sign/1 -> Product/1
  Product/1 -> dPed-comp/1
  1-D Lookup Table1/1 -> Sign/1
  Rb_rps/1 -> Sum5/1
  r_ideal_delay/1 -> Discrete-Time Integrator2/1, Sum1/1, yaw rate/1
  Discrete-Time Integrator2/1 -> Sum2/1
  Discrete-Time Integrator/1 -> Sum2/2
  Sum2/1 -> Gain1/1
  Sum3/1 -> Sum4/2
  Sum4/1 -> Product/2
  Gain1/1 -> Sum4/1
  [Vabs] -> 1-D Lookup Table1/1
  Constant2/1 -> 1-D Lookup Table1/2
  Vabs_kts/1 -> [Vabs]
  Sum5/1 -> Discrete-Time Integrator/1, Sum1/2, yaw rate/2
  Constant3/1 -> Sum5/2
  Enable_FB/1 -> Product2/1, Product1/1
  Sum1/1 -> error/1, Product1/2  "r_err"
  Discrete-Time Integrator1/1 -> Sum3/3
  Product2/1 -> Discrete-Time Integrator1/1
  Gain2/1 -> Sum/1
  TR/1 -> Sum/2

== system ground_test_EMF_new/EMF CLAWS/ACAH EMF1/Inner Loop - ACAH/[Heave] Cmd Filter // Inv Model ==
  note: Inverse Model
  note: Command Filter
  w_cmd (ft/s) : Inport
  Vabs_kts : Inport  Port=2
  1-D Lookup Table : Lookup_n-D  NumberOfTableDimensions=1  BreakpointsForDimension1=EMF.VTAB  BeginIndexSearchUsingPreviousIndexResult=on  TableSource=Input port  Table=tanh([-5:5])  ExtrapMethod=Clip  InternalRulePriority=Speed  OutDataTypeStr=single  RndMeth=Simplest
      settings: InputPortMap=u0,p221
  1-D Lookup Table1 : Lookup_n-D  NumberOfTableDimensions=1  BreakpointsForDimension1=EMF.VTAB  BeginIndexSearchUsingPreviousIndexResult=on  TableSource=Input port  Table=tanh([-5:5])  ExtrapMethod=Clip  InternalRulePriority=Speed  OutDataTypeStr=single  RndMeth=Simplest
      settings: InputPortMap=u0,p221
  Bus Creator : BusCreator  Inputs=2
  Constant : Constant  Value=EMF.wTau  OutDataTypeStr=single
  Constant1 : Constant  Value=EMF.Zw  OutDataTypeStr=single
  Constant3 : Constant  Value=EMF.Zcol  OutDataTypeStr=single
  Delay : Delay  DelayLength=EMF.HeaveDelay/framePeriod_s
  Delay1 : Delay  DelayLength=EMF.HeaveDelay/framePeriod_s
  Discrete-Time Integrator : DiscreteIntegrator  SampleTime=-1  OutDataTypeStr=single  ICPrevOutput=DiscIntNeverNeededParam  ICPrevScaledInput=DiscIntNeverNeededParam
  Divide : Product  Inputs=*/  OutDataTypeStr=single
  Divide1 : Product  Inputs=*/  OutDataTypeStr=single
  Product3 : Product
  Sum : Sum  Inputs=|+-
  Sum2 : Sum  Inputs=|+-
  col_ff : Outport
  w_ideal : Outport  Port=2
  cmdFilValues : Outport  Port=3
  wires:
  [wdot_ideal] -> Delay/1  "wdot_ideal"
  [w_ideal] -> Delay1/1  "Vz_ideal"
  Bus Creator/1 -> cmdFilValues/1
  Divide/1 -> Discrete-Time Integrator/1, Sum2/1, [wdot_ideal]  "wdot_ideal"
  Discrete-Time Integrator/1 -> w_ideal/1, [w_ideal], Product3/2, Sum/2  "w_ideal"
  Sum/1 -> Divide/1
  w_cmd (ft/s)/1 -> Sum/1
  Sum2/1 -> Divide1/1
  Constant/1 -> Divide/2
  Product3/1 -> Sum2/2
  Divide1/1 -> col_ff/1
  [Vabs] -> 1-D Lookup Table/1
  Constant1/1 -> 1-D Lookup Table/2
  1-D Lookup Table/1 -> Product3/1
  [Vabs] -> 1-D Lookup Table1/1
  Constant3/1 -> 1-D Lookup Table1/2
  1-D Lookup Table1/1 -> Divide1/2
  Vabs_kts/1 -> [Vabs]
  Delay/1 -> Bus Creator/1  "Vzdot_filtered"
  Delay1/1 -> Bus Creator/2  "Vz_filtered"

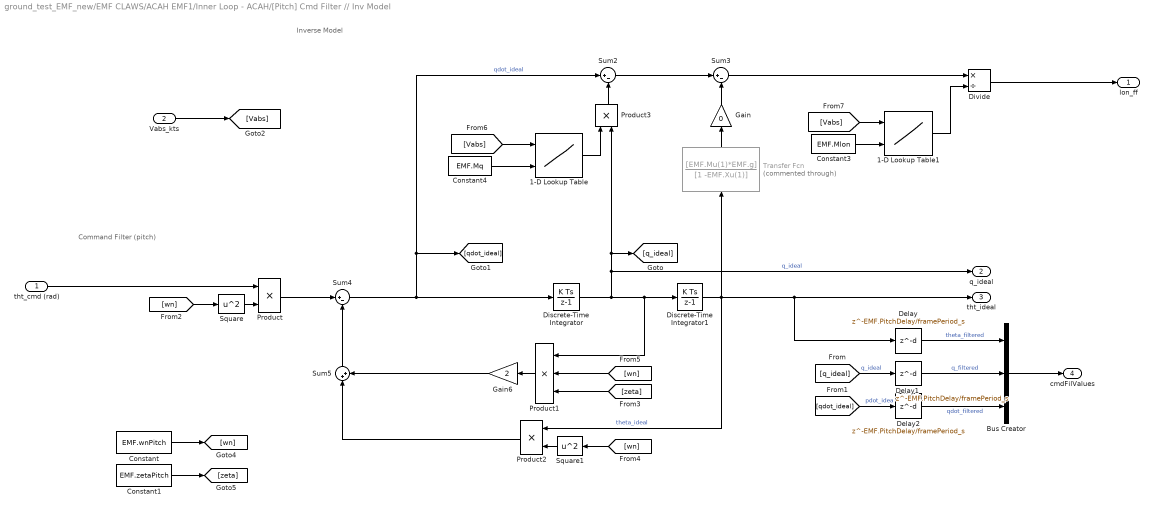
== system ground_test_EMF_new/EMF CLAWS/ACAH EMF1/Inner Loop - ACAH/[Pitch] Cmd Filter // Inv Model ==
  note: Command Filter (pitch)
  note: Inverse Model
  tht_cmd (rad) : Inport
  Vabs_kts : Inport  Port=2
  1-D Lookup Table : Lookup_n-D  NumberOfTableDimensions=1  BreakpointsForDimension1=EMF.VTAB  BeginIndexSearchUsingPreviousIndexResult=on  TableSource=Input port  Table=tanh([-5:5])  ExtrapMethod=Clip  InternalRulePriority=Speed  RndMeth=Simplest
      settings: InputPortMap=u0,p221
  1-D Lookup Table1 : Lookup_n-D  NumberOfTableDimensions=1  BreakpointsForDimension1=EMF.VTAB  BeginIndexSearchUsingPreviousIndexResult=on  TableSource=Input port  Table=tanh([-5:5])  ExtrapMethod=Clip  InternalRulePriority=Speed  RndMeth=Simplest
      settings: InputPortMap=u0,p221
  Bus Creator : BusCreator  Inputs=3
  Constant : Constant  Value=EMF.wnPitch
  Constant1 : Constant  Value=EMF.zetaPitch
  Constant3 : Constant  Value=EMF.Mlon
  Constant4 : Constant  Value=EMF.Mq
  Delay : Delay  DelayLength=EMF.PitchDelay/framePeriod_s
  Delay1 : Delay  DelayLength=EMF.PitchDelay/framePeriod_s
  Delay2 : Delay  DelayLength=EMF.PitchDelay/framePeriod_s
  Discrete-Time Integrator : DiscreteIntegrator  SampleTime=-1  ICPrevOutput=DiscIntNeverNeededParam  ICPrevScaledInput=DiscIntNeverNeededParam
  Discrete-Time Integrator1 : DiscreteIntegrator  SampleTime=-1  ICPrevOutput=DiscIntNeverNeededParam  ICPrevScaledInput=DiscIntNeverNeededParam
  Divide : Product  Inputs=*/
  Gain : Gain  Gain=0
  Gain6 : Gain  Gain=2
  Product : Product
  Product1 : Product  Inputs=3
  Product2 : Product
  Product3 : Product
  Square : Math  Operator=square
  Square1 : Math  Operator=square
  Sum2 : Sum  Inputs=|+-
  Sum3 : Sum  Inputs=|+-
  Sum4 : Sum  Inputs=|+-
  Sum5 : Sum  Inputs=|++
  Transfer Fcn : TransferFcn  Commented=through  Numerator=[EMF.Mu(1)*EMF.g]  Denominator=[1 -EMF.Xu(1)]
  lon_ff : Outport
  q_ideal : Outport  Port=2
  tht_ideal : Outport  Port=3
  cmdFilValues : Outport  Port=4
  wires:
  [q_ideal] -> Delay1/1  "q_ideal"
  [qdot_ideal] -> Delay2/1  "pdot_idea"
  Bus Creator/1 -> cmdFilValues/1
  Sum2/1 -> Sum3/1
  tht_cmd (rad)/1 -> Product/1
  Transfer Fcn/1 -> Gain/1
  [wn] -> Product1/2
  Product1/1 -> Gain6/1
  [zeta] -> Product1/3
  Constant1/1 -> [zeta]
  Gain6/1 -> Sum5/2
  Product/1 -> Sum4/1
  Constant/1 -> [wn]
  Square1/1 -> Product2/2
  [wn] -> Square1/1
  Square/1 -> Product/2
  Discrete-Time Integrator/1 -> Product3/2, [q_ideal], q_ideal/1, Discrete-Time Integrator1/1, Product1/1  "q_ideal"
  [wn] -> Square/1
  Discrete-Time Integrator1/1 -> Delay/1, tht_ideal/1, Transfer Fcn/1, Product2/1  "theta_ideal"
  Sum4/1 -> Discrete-Time Integrator/1, [qdot_ideal], Sum2/1  "qdot_ideal"
  Sum5/1 -> Sum4/2
  Product2/1 -> Sum5/1
  1-D Lookup Table/1 -> Product3/1
  Product3/1 -> Sum2/2
  Sum3/1 -> Divide/1
  Divide/1 -> lon_ff/1
  Gain/1 -> Sum3/2
  [Vabs] -> 1-D Lookup Table/1
  Constant4/1 -> 1-D Lookup Table/2
  Constant3/1 -> 1-D Lookup Table1/2
  1-D Lookup Table1/1 -> Divide/2
  [Vabs] -> 1-D Lookup Table1/1
  Vabs_kts/1 -> [Vabs]
  Delay/1 -> Bus Creator/1  "theta_filtered"
  Delay1/1 -> Bus Creator/2  "q_filtered"
  Delay2/1 -> Bus Creator/3  "qdot_filtered"

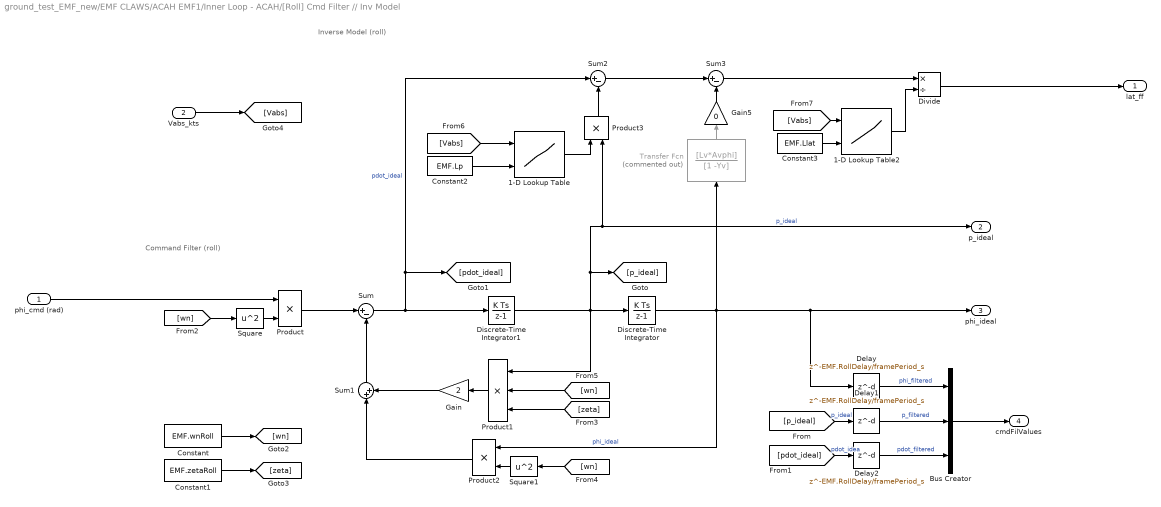
== system ground_test_EMF_new/EMF CLAWS/ACAH EMF1/Inner Loop - ACAH/[Roll] Cmd Filter // Inv Model ==
  note: Command Filter (roll)
  note: Inverse Model (roll)
  phi_cmd (rad) : Inport
  Vabs_kts : Inport  Port=2
  1-D Lookup Table : Lookup_n-D  NumberOfTableDimensions=1  BreakpointsForDimension1=EMF.VTAB  BeginIndexSearchUsingPreviousIndexResult=on  TableSource=Input port  Table=tanh([-5:5])  ExtrapMethod=Clip  InternalRulePriority=Speed  RndMeth=Simplest
      settings: InputPortMap=u0,p221
  1-D Lookup Table2 : Lookup_n-D  NumberOfTableDimensions=1  BreakpointsForDimension1=EMF.VTAB  BeginIndexSearchUsingPreviousIndexResult=on  TableSource=Input port  Table=tanh([-5:5])  ExtrapMethod=Clip  InternalRulePriority=Speed  RndMeth=Simplest
      settings: InputPortMap=u0,p221
  Bus Creator : BusCreator  Inputs=3
  Constant : Constant  Value=EMF.wnRoll
  Constant1 : Constant  Value=EMF.zetaRoll
  Constant2 : Constant  Value=EMF.Lp
  Constant3 : Constant  Value=EMF.Llat
  Delay : Delay  DelayLength=EMF.RollDelay/framePeriod_s
  Delay1 : Delay  DelayLength=EMF.RollDelay/framePeriod_s
  Delay2 : Delay  DelayLength=EMF.RollDelay/framePeriod_s
  Discrete-Time Integrator : DiscreteIntegrator  SampleTime=-1  ICPrevOutput=DiscIntNeverNeededParam  ICPrevScaledInput=DiscIntNeverNeededParam
  Discrete-Time Integrator1 : DiscreteIntegrator  SampleTime=-1  ICPrevOutput=DiscIntNeverNeededParam  ICPrevScaledInput=DiscIntNeverNeededParam
  Divide : Product  Inputs=*/
  Gain : Gain  Gain=2
  Gain5 : Gain  Gain=0
  Product : Product
  Product1 : Product  Inputs=3
  Product2 : Product
  Product3 : Product
  Square : Math  Operator=square
  Square1 : Math  Operator=square
  Sum : Sum  Inputs=|+-
  Sum1 : Sum  Inputs=|++
  Sum2 : Sum  Inputs=|+-
  Sum3 : Sum  Inputs=|+-
  Transfer Fcn : TransferFcn  Commented=on  Numerator=[Lv*Avphi]  Denominator=[1 -Yv]
  lat_ff : Outport
  p_ideal : Outport  Port=2
  phi_ideal : Outport  Port=3
  cmdFilValues : Outport  Port=4
  wires:
  Transfer Fcn/1 -> Gain5/1
  Sum2/1 -> Sum3/1
  Sum3/1 -> Divide/1
  Bus Creator/1 -> cmdFilValues/1
  [pdot_ideal] -> Delay2/1  "pdot_idea"
  [p_ideal] -> Delay1/1  "p_ideal"
  Product3/1 -> Sum2/2
  Divide/1 -> lat_ff/1
  Product2/1 -> Sum1/1
  Sum1/1 -> Sum/2
  Product/1 -> Sum/1
  Sum/1 -> Discrete-Time Integrator1/1, [pdot_ideal], Sum2/1  "pdot_ideal"
  Gain/1 -> Sum1/2
  Discrete-Time Integrator/1 -> Product2/1, Transfer Fcn/1, Delay/1, phi_ideal/1  "phi_ideal"
  Discrete-Time Integrator1/1 -> Discrete-Time Integrator/1, Product1/1, [p_ideal], Product3/2, p_ideal/1  "p_ideal"
  phi_cmd (rad)/1 -> Product/1
  Gain5/1 -> Sum3/2
  Square/1 -> Product/2
  Constant/1 -> [wn]
  [wn] -> Square/1
  Constant1/1 -> [zeta]
  [wn] -> Square1/1
  Square1/1 -> Product2/2
  [zeta] -> Product1/3
  [wn] -> Product1/2
  Product1/1 -> Gain/1
  Constant2/1 -> 1-D Lookup Table/2
  1-D Lookup Table/1 -> Product3/1
  Constant3/1 -> 1-D Lookup Table2/2
  1-D Lookup Table2/1 -> Divide/2
  Vabs_kts/1 -> [Vabs]
  [Vabs] -> 1-D Lookup Table/1
  [Vabs] -> 1-D Lookup Table2/1
  Delay/1 -> Bus Creator/1  "phi_filtered"
  Delay1/1 -> Bus Creator/2  "p_filtered"
  Delay2/1 -> Bus Creator/3  "pdot_filtered"

== system ground_test_EMF_new/EMF CLAWS/ACAH EMF1/Inner Loop - ACAH/[Yaw] Cmd Filter // Inv Model ==
  note: Command Filter
  note: Inverse Model
  r_cmd (rad/s) : Inport
  Vabs_kts : Inport  Port=2
  1-D Lookup Table1 : Lookup_n-D  NumberOfTableDimensions=1  BreakpointsForDimension1=EMF.VTAB  BeginIndexSearchUsingPreviousIndexResult=on  TableSource=Input port  Table=tanh([-5:5])  ExtrapMethod=Clip  InternalRulePriority=Speed  OutDataTypeStr=single  RndMeth=Simplest
      settings: InputPortMap=u0,p221
  1-D Lookup Table2 : Lookup_n-D  NumberOfTableDimensions=1  BreakpointsForDimension1=EMF.VTAB  BeginIndexSearchUsingPreviousIndexResult=on  TableSource=Input port  Table=tanh([-5:5])  ExtrapMethod=Clip  InternalRulePriority=Speed  OutDataTypeStr=single  RndMeth=Simplest
      settings: InputPortMap=u0,p221
  Bus Creator : BusCreator  Inputs=2
  Constant : Constant  Value=EMF.rTau  OutDataTypeStr=single
  Constant2 : Constant  Value=EMF.Nr  OutDataTypeStr=single
  Constant3 : Constant  Value=EMF.Nped  OutDataTypeStr=single
  Delay : Delay  DelayLength=EMF.YawDelay/framePeriod_s
  Delay1 : Delay  DelayLength=EMF.YawDelay/framePeriod_s
  Discrete-Time Integrator : DiscreteIntegrator  SampleTime=-1  OutDataTypeStr=single  ICPrevOutput=DiscIntNeverNeededParam  ICPrevScaledInput=DiscIntNeverNeededParam
  Divide : Product  Inputs=*/  OutDataTypeStr=single
  Divide1 : Product  Inputs=*/  OutDataTypeStr=single
  Product3 : Product
  Sum : Sum  Inputs=|+-
  Sum2 : Sum  Inputs=|+-
  ped_ff : Outport
  r_ideal : Outport  Port=2
  cmdFilValues : Outport  Port=3
  wires:
  [rdot_ideal] -> Delay/1  "rdot_ideal"
  Bus Creator/1 -> cmdFilValues/1
  [r_ideal] -> Delay1/1  "r_ideal"
  Divide/1 -> Discrete-Time Integrator/1, Sum2/1, [rdot_ideal]  "rdot_ideal"
  Sum2/1 -> Divide1/1
  r_cmd (rad/s)/1 -> Sum/1
  Sum/1 -> Divide/1
  Discrete-Time Integrator/1 -> Product3/2, Sum/2, r_ideal/1, [r_ideal]  "r_ideal"
  Constant/1 -> Divide/2
  Product3/1 -> Sum2/2
  Divide1/1 -> ped_ff/1
  [Vabs] -> 1-D Lookup Table1/1
  Constant2/1 -> 1-D Lookup Table1/2
  Constant3/1 -> 1-D Lookup Table2/2
  [Vabs] -> 1-D Lookup Table2/1
  1-D Lookup Table1/1 -> Product3/1
  1-D Lookup Table2/1 -> Divide1/2
  Vabs_kts/1 -> [Vabs]
  Delay/1 -> Bus Creator/1  "rdot_filtered"
  Delay1/1 -> Bus Creator/2  "r_filtered"

== system ground_test_EMF_new/EMF CLAWS/ACAH EMF1/OnGroundController/Get ACAH Commands1 ==
  StickInputs : Inport
  Constant : Constant  Value=-1
  Constant1 : Constant
  Constant2 : Constant  Value=0
  Demux : Demux
  Gain{,1..3} (4 alike) : Gain  Gain=0
  Mux : Mux
  Saturation{,1..3} (4 alike) : Saturate  UpperLimit=1  LowerLimit=-1
  remap throttle to RPM : MATLAB Function  TreatAsAtomicUnit=on
  rotor speed : Constant  Value=mean(InitCond.TrimInputs)*2
  cmdsACAH : Outport
  throttleOmega : Outport  Port=2
  wires:
  StickInputs/1 -> Demux/1
  Demux/1 -> Saturation/1
  Demux/2 -> Saturation1/1
  Demux/3 -> Saturation2/1
  Demux/4 -> Saturation3/1
  Saturation/1 -> Gain/1
  Saturation1/1 -> Gain1/1
  Saturation3/1 -> Gain3/1
  Gain3/1 -> Mux/4
  Mux/1 -> cmdsACAH/1
  Gain1/1 -> Mux/3
  Gain/1 -> Mux/2
  Gain2/1 -> Mux/1
  rotor speed/1 -> remap throttle to RPM/5(out_max)
  Constant2/1 -> remap throttle to RPM/4(out_min)
  Constant/1 -> remap throttle to RPM/2(in_min)
  remap throttle to RPM/1(raw_out) -> throttleOmega/1  "PWM_cont"
  Saturation2/1 -> remap throttle to RPM/1(norm_in), Gain2/1
  Constant1/1 -> remap throttle to RPM/3(in_max)

== system ground_test_EMF_new/EMF CLAWS/ACAH EMF1/OnGroundController/OL rotor speeds from throttle ==
  throttleOmega : Inport
  Gain : Gain  Gain=InitCond.Omega1_rps/mean([InitCond.Omega1_rps, InitCond.Omega2_rps])
  Gain1 : Gain  Gain=InitCond.Omega2_rps/mean([InitCond.Omega1_rps, InitCond.Omega2_rps])
  Gain2 : Gain  Gain=InitCond.Omega3_rps/mean([InitCond.Omega1_rps, InitCond.Omega2_rps])
  Gain3 : Gain  Gain=InitCond.Omega4_rps/mean([InitCond.Omega1_rps, InitCond.Omega2_rps])
  Mux2 : Mux
  Omegas_rps : Outport
  wires:
  throttleOmega/1 -> Gain3/1, Gain2/1, Gain1/1, Gain/1
  Gain/1 -> Mux2/1
  Gain1/1 -> Mux2/2
  Gain2/1 -> Mux2/3
  Gain3/1 -> Mux2/4
  Mux2/1 -> Omegas_rps/1

== system ground_test_EMF_new/EMF CLAWS/ACAH EMF1/Remap Rotor Speeds to PWM/Rotor Speed Saturation ==
  Rotor Speeds : Inport
  Compare To Constant7 : simulink/Logic and Bit Operations/Compare To Constant  relop=<  const=AircraftModel.MinOmegaLimit(1)  OutDataTypeStr=boolean
  Compare To Constant8 : simulink/Logic and Bit Operations/Compare To Constant  relop=>  const=AircraftModel.MaxOmegaLimit(1)  OutDataTypeStr=boolean
  Logical Operator4 : Logic  Operator=OR  AllPortsSameDT=off  OutDataTypeStr=boolean
  Saturation4 : Saturate  UpperLimit=AircraftModel.MaxOmegaLimit(1)  LowerLimit=AircraftModel.MinOmegaLimit(1)
  OmegaSaturationFlags : Outport
  Saturated Rotor Speeds : Outport  Port=2
  wires:
  Saturation4/1 -> Saturated Rotor Speeds/1
  Rotor Speeds/1 -> Compare To Constant8/1, Compare To Constant7/1, Saturation4/1
  Logical Operator4/1 -> OmegaSaturationFlags/1
  Compare To Constant8/1 -> Logical Operator4/1
  Compare To Constant7/1 -> Logical Operator4/2

== matlab function ground_test_EMF_new/command selection/throttle_norm/remap ==
  data: raw_in input; norm_out output; in_min input; in_max input; out_min input; out_max input
function norm_out = remap(raw_in,in_min,in_max,out_min,out_max)
norm_out = (raw_in - in_min) * (out_max - out_min)/(in_max-in_min) + out_min;

== matlab function ground_test_EMF_new/command selection/yaw_norm_deadband/remap_with_deadband ==
  data: raw_in input; norm_out output; in_min input; in_max input; out_min input; out_max input; deadband input
function norm_out = remap_deadband(raw_in, in_min, in_max, out_min, out_max, deadband)
in_avg = (in_min + in_max) / 2;
out_avg = (out_min + out_max) / 2;

in_deadband_range = (in_max - in_min) * deadband / 2;
in_deadband_low = in_avg - in_deadband_range;
in_deadband_hi = in_avg + in_deadband_range;

if raw_in < in_deadband_low
    norm_out = (raw_in - in_deadband_low) .* (out_max - out_avg)./(in_deadband_low - in_min) + out_avg;
elseif raw_in > in_deadband_low && raw_in < in_deadband_hi
    norm_out = out_avg;
else
    norm_out = (raw_in - in_deadband_hi) .* (out_max - out_avg)./(in_max - in_deadband_hi) + out_avg;
end

== matlab function ground_test_EMF_new/EMF CLAWS/ACAH EMF1/OnGroundController/Get ACAH Commands1/remap throttle to RPM ==
  data: norm_in input; raw_out output; in_min input; in_max input; out_min input; out_max input
function raw_out = remap(norm_in,in_min,in_max,out_min,out_max)
raw_out = (norm_in - in_min) * (out_max - out_min)/(in_max-in_min) + out_min;

== matlab function ground_test_EMF_new/EMF CLAWS/ACAH EMF1/Remap Rotor Speeds to PWM/remap ==
  data: norm_in input; raw_out output; in_min input; in_max input; out_min input; out_max input
function raw_out = arrayremap(norm_in,in_min,in_max,out_min,out_max)
raw_out = norm_in*0;
for i = 1:length(norm_in)
raw_out(i) = (norm_in(i) - in_min(i)) * (out_max(i) - out_min(i))/(in_max(i)-in_min(i)) + out_min(i);
end
end

== matlab function ground_test_EMF_new/EMF CLAWS/PWM to Linear Model Inputs/remap ==
  data: norm_in input; raw_out output; in_min input; in_max input; out_min input; out_max input
function raw_out = arrayremap(norm_in,in_min,in_max,out_min,out_max)
raw_out = norm_in*0;
for i = 1:length(norm_in)
raw_out(i) = (norm_in(i) - in_min(i)) * (out_max(i) - out_min(i))/(in_max(i)-in_min(i)) + out_min(i);
end
end

== matlab function ground_test_EMF_new/command selection/e-stop/remap ==
  data: raw_in input; norm_out output; in_min input; in_max input; out_min input; out_max input
function norm_out = remap(raw_in,in_min,in_max,out_min,out_max)
norm_out = (raw_in - in_min) * (out_max - out_min)/(in_max-in_min) + out_min;

== matlab function ground_test_EMF_new/command selection/mode_norm/remap ==
  data: raw_in input; norm_out output; in_min input; in_max input; out_min input; out_max input
function norm_out = remap(raw_in,in_min,in_max,out_min,out_max)
norm_out = (raw_in - in_min) * (out_max - out_min)/(in_max-in_min) + out_min;

== matlab function ground_test_EMF_new/remap ==
  data: raw_in input; norm_out output; in_min input; in_max input; out_min input; out_max input
function norm_out = remap(raw_in,in_min,in_max,out_min,out_max)
norm_out = (raw_in - in_min) * (out_max - out_min)/(in_max-in_min) + out_min;
